simulink model "Rack_assist"  (R2024a)
settings: Solver=VariableStepAuto  StartTime=0.0  StopTime=10.0  RelTol=1e-3
libraries: fl_lib x12, nesl_utility x9, sdl_lib x3, ee_lib x1
settings Model: Creator=jesus  LastModifiedBy=kamal

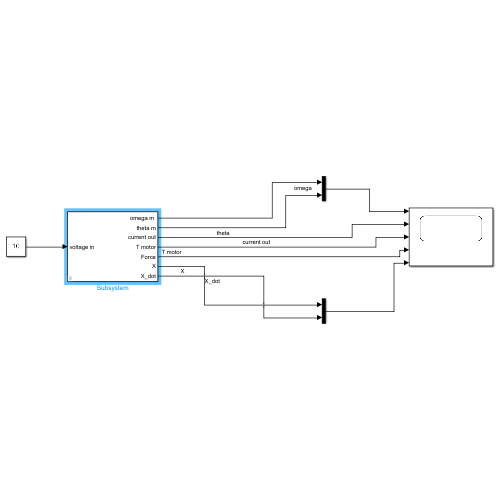
[thumbnail: Simulink's stored preview of the top-level diagram]
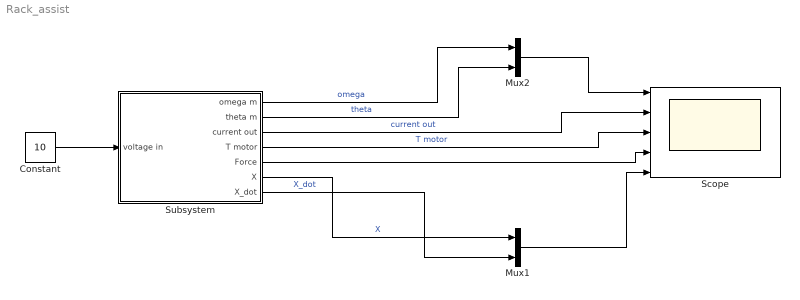
== system Rack_assist ==
  Constant : Constant  Value=10
  Mux1 : Mux  Inputs=2
  Mux2 : Mux  Inputs=2
  Scope : Scope  NumInputPorts=5
  Subsystem : Subsystem  mask{Ra=0.1, La=0.1e-3, Ke=0.01, Im=30, Bm=0.003339, Jm=0.0004704, mr=2, Br=100, rp=10e-3}
      mask prompts: Ra "Armature resistance"; La "Armature inductance"; Ke "Back Emf costant"; Im "Rack & pinion ratio"; Bm "motor friction"; Jm "motor inertia"; mr "Rack mass"; Br "Rack friction coefficient"; rp "pinion radius"
  wires:
  Constant/1 -> Subsystem/1(voltage in)
  Subsystem/1("omega m ") -> Mux2/1  "omega"
  Subsystem/2(theta m) -> Mux2/2  "theta"
  Subsystem/3(current out) -> Scope/2  "current out"
  Subsystem/6(X) -> Mux1/1  "X"
  Subsystem/7(X_dot) -> Mux1/2  "X_dot"
  Mux1/1 -> Scope/5
  Mux2/1 -> Scope/1
  Subsystem/4(T motor) -> Scope/3  "T motor"
  Subsystem/5(Force) -> Scope/4

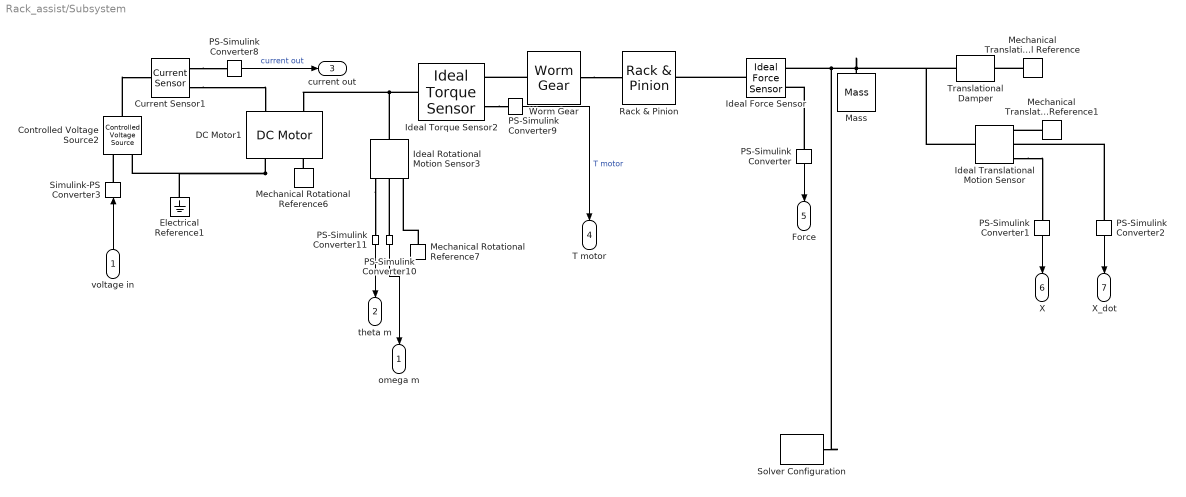
== system Rack_assist/Subsystem ==
  voltage in : Inport
  Controlled Voltage Source2 : fl_lib/Electrical/Electrical Sources/Controlled Voltage Source
  Current Sensor1 : fl_lib/Electrical/Electrical Sensors/Current Sensor
  DC Motor1 : ee_lib/Electromechanical/Brushed Motors/DC Motor  field_option=ee.enum.field_option.pm  Rf=100 Ohm  Lf=1 H  Laf=0.15 H  If0=0 A  parameterization=ee.enum.dcparam_option.circuit_param  Ra=Ra Ohm  La=La H  emf_or_torque=ee.enum.emf_or_torque.kv  Kv=Ke V/rpm  Ki=6.876e-4 N*m/A  T_stall=0.24e-3 N*m  w_max=19100 rpm  w_rated=15000 rpm  P_rated=0.08 W  V_rated=1.5 V  lam_param=ee.enum.lam_param.damping  i_noload=0 A  V_i_noload=1.5 V  J=Jm kg*m^2  lam=Bm N*m*s/rad  speed0=0 rpm  enable_fault_armature=simscape.enum.onoff.off  rev_faulted=1 / 3  G_faulted_armature=1e-5 S  fault_trigger_armature=ee.enum.faults.faultTrigger.temporal  t_fault_armature=1 s  max_permissible_current_armature=inf A  t_fail_on_current_armature=1 s  enable_fault_field=simscape.enum.onoff.off  G_faulted_field=1e-5 S  fault_trigger_field=ee.enum.faults.faultTrigger.temporal  t_fault_field=1 s  max_permissible_current_field=inf A  t_fail_on_current_field=1 s  fault_action=simscape.enum.assert.action.none  alpha=3.93e-3 1/K  Tmeas=25 degC  thermal_mass=100 J/K  initial_temperature=25 degC
  Electrical Reference1 : fl_lib/Electrical/Electrical Elements/Electrical Reference
  Ideal Force Sensor : fl_lib/Mechanical/Mechanical Sensors/Ideal Force Sensor
  Ideal Rotational Motion Sensor3 : fl_lib/Mechanical/Mechanical Sensors/Ideal Rotational Motion Sensor  reference=foundation.enum.MeasurementReference.difference  acceleration_port=false  velocity_port=true  position_port=true  wrap_angle=false  offset=0 rad
  Ideal Torque Sensor2 : fl_lib/Mechanical/Mechanical Sensors/Ideal Torque Sensor
  Ideal Translational Motion Sensor : fl_lib/Mechanical/Mechanical Sensors/Ideal Translational Motion Sensor  reference=foundation.enum.MeasurementReference.difference  acceleration_port=false  velocity_port=true  position_port=true  offset=0 m
  Mass : fl_lib/Mechanical/Translational Elements/Mass  mass=mr kg  num_ports=foundation.enum.numPorts2.one  v_specify=off  v_priority=High  v=0 m/s  v_nominal_specify=off  v_nominal_value=1  v_nominal_unit=m/s  f_specify=off  f_priority=None  f=0 N  f_nominal_specify=off  f_nominal_value=1  f_nominal_unit=N
  Mechanical Rotational Reference6 : fl_lib/Mechanical/Rotational Elements/Mechanical Rotational Reference
  Mechanical Rotational Reference7 : fl_lib/Mechanical/Rotational Elements/Mechanical Rotational Reference
  Mechanical Translational Reference : fl_lib/Mechanical/Translational Elements/Mechanical Translational Reference
  Mechanical Translational Reference1 : fl_lib/Mechanical/Translational Elements/Mechanical Translational Reference
  PS-Simulink Converter{,1..2,8..11} (7 alike) : nesl_utility/PS-Simulink Converter  PhysicalDomain=network_engine_domain  SubClassName=ps_output  LeftPortType=input  RightPortType=output  PseudoPeriodic=off  Frequencies=[]  VectorFormat=inherit  Unit=inherit  AffineConversion=off
  Rack & Pinion : sdl_lib/Gears/Rotational- Translational/Rack & Pinion  param=sdl.enum.rackPinionParameters.radius  radius=rp m  n_teeth=20  x_tooth=5 mm  rack_direction_sign=sdl.enum.pinionDirection.positive  friction_model=sdl.enum.gear_friction.none  efficiency=0.8  temperature_TLU=[280, 300, 320] K  efficiency_TLU=[.95, .9, .85]  pwr_thr=0.001 W  mu_visc_P=0 N*m*s/rad  mu_visc_R=0 N*s/m  thermal_mass=50 J/K  temperature_specify=off  temperature_priority=High  temperature=300 K  temperature_nominal_specify=off  temperature_nominal_value=1  temperature_nominal_unit=K
      settings: InternalSimscapePortConfiguration="{\"Bottom\":[],\"Left\":[{\"id\":\"P\",\"label\":\"P\",\"type\":\"foundation.mechanical.rotational.rotational\"}],\"Right\":[{\"id\":\"R\",\"label\":\"R\",\"type\":\"foundation.mechanical.translational.translational\"}],\"Top\":[]}"
  Simulink-PS Converter3 : nesl_utility/Simulink-PS Converter  PhysicalDomain=network_engine_domain  SubClassName=ps_input  LeftPortType=input  RightPortType=output  PseudoPeriodic=off  Frequencies=[]  NoiseDistribution=none  NoiseParameters=[]  Unit=1  AffineConversion=off  FilteringAndDerivatives=provide  SimscapeFilterOrder=1  InputFilterTimeConstant=0.001  UdotUserProvided=0
  Solver Configuration : nesl_utility/Solver Configuration  PhysicalDomain=network_engine_domain  SubClassName=solver  LeftPortType=input  RightPortType=generic  Tones=[]  Harmonics=[]  SimulateNoise=off  Profile=off  UseLocalSampling=off  EnableSwitchedLinearOptims=on  FrequencyDomain=off  UseCCode=off  RelTol=0.001  AbsTol=0.001  MinStep=1e-09  ToWorkspace=off  RevertToSquareIcSolve=off  NumHomotopyIterations=100  PhasorMode=off  PhasorModeNumHarmonics=1  ConsistencySolver=NEWTON_XTOL_AFTER_FTOL  IndexReductionMethod=DerivativeReplacement  DoDC=off  ResidualTolerance=1e-09  ConsistencyTolSource=GLOBAL  ConsistencyAbsTol=0.001  ConsistencyRelTol=0.001  ConsistencyTolFactor=0.001  UseLocalSolver=off  LocalSolverChoice=NE_BACKWARD_EULER_ADVANCER  ResolveIndetEquations=on  FunctionEvalNumThread=1  LocalSolverSampleTime=0.001  DoFixedCost=off  MaxNonlinIter=3  MaxModeIter=2  ComputeImpulses=off  ImpulseIterations=2  LinearAlgebra=auto  LinearAlgebraNumThread=0  EquationFormulation=NE_TIME_EF  DelaysMemoryBudget=1024  AutomaticFiltering=on  FilteringTimeConstant=0.001  PartitionStorageMethod=AS_NEEDED  PartitionMemoryBudget=1024  PartitionMethod=ROBUST  MultibodyUseLocalSolver=off  MultibodyLocalSolverChoice=ODE1  MultibodyLocalSolverSampleTime=0.001
  Translational Damper : sdl_lib/Couplings & Drives/Springs & Dampers/Translational Damper  D=Br N*s/m  enable_faults=simscape.enum.onoff.off  b_fault=1e6 N*s/m  fault_trigger=simscape.fault.triggertype.external  acceleration_limit=100 m/s^2  shock_limit=1  thermal_port=simscape.enum.thermaleffects.omit  thermal_mass=50 kJ/K  temperature_specify=off  temperature_priority=High  temperature=300 K  temperature_nominal_specify=off  temperature_nominal_value=1  temperature_nominal_unit=K
  Worm Gear : sdl_lib/Gears/Worm Gear  ratio=Im  thread_type=sdl.enum.handedness.right  friction_model=sdl.enum.gear_friction.none  friction_parameterization=sdl.enum.efficiency_geometry.geometry  pr_ang=17.5 deg  lead_ang=20 deg  fr_coeff=0.08  eff_wg=0.74  eff_gw=0.65  temperature_TLU=[280, 300, 320] K  efficiency_wg_TLU=[.75, .65, .6]  efficiency_gw_TLU=[.5, .45, .4]  pwr_thr=0.001 W  mu_visc=[0, 0] N*m*s/rad  thermal_mass=50 J/K  temperature_specify=off  temperature_priority=High  temperature=300 K  temperature_nominal_specify=off  temperature_nominal_value=1  temperature_nominal_unit=K
      settings: InternalSimscapePortConfiguration="{\"Bottom\":[],\"Left\":[{\"id\":\"W\",\"label\":\"W\",\"type\":\"foundation.mechanical.rotational.rotational\"}],\"Right\":[{\"id\":\"G\",\"label\":\"G\",\"type\":\"foundation.mechanical.rotational.rotational\"}],\"Top\":[]}"
  "omega m " : Outport
  theta m : Outport  Port=2
  current out : Outport  Port=3
  T motor : Outport  Port=4
  Force : Outport  Port=5
  X : Outport  Port=6
  X_dot : Outport  Port=7
  wires:
  PS-Simulink Converter10/1 -> "omega m "/1
  PS-Simulink Converter8/1 -> current out/1  "current out"
  PS-Simulink Converter11/1 -> theta m/1
  PS-Simulink Converter9/1 -> T motor/1  "T motor"
  voltage in/1 -> Simulink-PS Converter3/1
  PS-Simulink Converter/1 -> Force/1
  PS-Simulink Converter1/1 -> X/1
  PS-Simulink Converter2/1 -> X_dot/1
  connections:
  Ideal Torque Sensor2/RConn2 -- PS-Simulink Converter9/LConn1
  Mechanical Rotational Reference7/LConn1 -- Ideal Rotational Motion Sensor3/RConn1
  Ideal Torque Sensor2/LConn1 -- DC Motor1/LConn2 -- Ideal Rotational Motion Sensor3/LConn1
  Current Sensor1/RConn1 -- PS-Simulink Converter8/LConn1
  PS-Simulink Converter10/LConn1 -- Ideal Rotational Motion Sensor3/RConn2
  Ideal Rotational Motion Sensor3/RConn3 -- PS-Simulink Converter11/LConn1
  Simulink-PS Converter3/RConn1 -- Controlled Voltage Source2/RConn1
  Controlled Voltage Source2/LConn1 -- Current Sensor1/LConn1
  Current Sensor1/RConn2 -- DC Motor1/LConn1
  Mechanical Rotational Reference6/LConn1 -- DC Motor1/RConn2
  DC Motor1/RConn1 -- Controlled Voltage Source2/RConn2 -- Electrical Reference1/LConn1
  Ideal Force Sensor/LConn1 -- Rack & Pinion/RConn1
  Worm Gear/LConn1 -- Ideal Torque Sensor2/RConn1
  Worm Gear/RConn1 -- Rack & Pinion/LConn1
  Mass/LConn1 -- Ideal Translational Motion Sensor/LConn1 -- Translational Damper/LConn1 -- Solver Configuration/RConn1 -- Ideal Force Sensor/RConn1
  Mechanical Translational Reference/LConn1 -- Translational Damper/RConn1
  PS-Simulink Converter/LConn1 -- Ideal Force Sensor/RConn2
  Mechanical Translational Reference1/LConn1 -- Ideal Translational Motion Sensor/RConn1
  Ideal Translational Motion Sensor/RConn3 -- PS-Simulink Converter1/LConn1
  PS-Simulink Converter2/LConn1 -- Ideal Translational Motion Sensor/RConn2
